simulink library "hamilton"  (R2023a)
settings: Solver=VariableStepAuto  StartTime=0.0  StopTime=10.0  RelTol=1e-3
undefined symbols (not defined in the file): b, d, g, J1, J2, J3, L, m
settings Model: Creator=Alex  LastModifiedBy=Alex

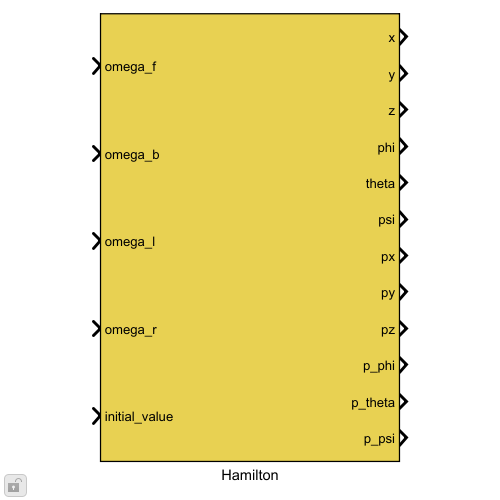
[thumbnail: Simulink's stored preview of the top-level diagram]
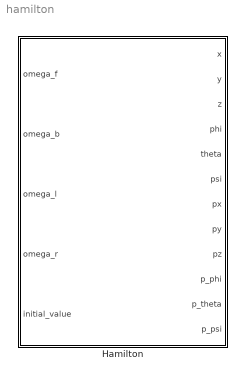
== system hamilton ==
  Hamilton : Subsystem

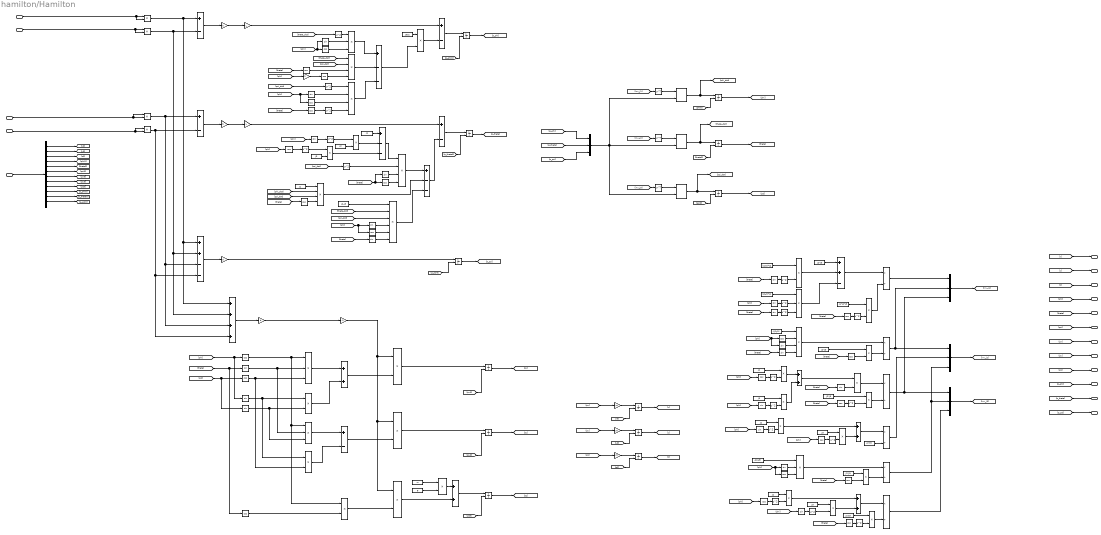
== system hamilton/Hamilton ==
  note: aefcascascxascx
  note: F_thrust
  note: Rotational generalized coordinates (positions)
  note: Translational generalized coordinates (positions)
  note: Translational momentum equations
  note: Rotational momentum equations
  note: Matrix J^(-1) computation
  omega_f : Inport
  omega_b : Inport  Port=2
  omega_l : Inport  Port=3
  omega_r : Inport  Port=4
  initial_value : Inport  Port=5
  Add{,1,3..4,11} (5 alike) : Sum  Inputs=+-
  Add{10,14,26..28} (5 alike) : Sum
  Add2 : Sum  Inputs=++--
  Add25 : Sum  Inputs=++-
  Add5 : Sum  Inputs=+--
  Add6 : Sum  Inputs=++++
  Add7 : Sum  Inputs=+--
  Add8 : Sum  Inputs=+--
  Constant1 : Constant  Value=J3-J2
  Constant2 : Constant  Value=J1
  Constant{22,26,28,31,34,36} (6 alike) : Constant  Value=J2*J3
  Constant23 : Constant  Value=(J1-J3)*J2
  Constant24 : Constant  Value=(J2-J3)*J1
  Constant25 : Constant  Value=J1*J2*J3
  Constant27 : Constant  Value=-(J2-J3)
  Constant{3,29,32,37} (4 alike) : Constant  Value=J2
  Constant{8,30,33,38} (4 alike) : Constant  Value=J3
  Constant35 : Constant  Value=-(J2-J3)
  Constant4 : Constant  Value=J1
  Constant5 : Constant  Value=J2-J3
  Constant6 : Constant  Value=m
  Constant7 : Constant  Value=g
  Cos{,1,3,5,7,53..55,58,60,63..64,66..67,69} (15 alike) : Trigonometry  Operator=cos
  Cos{4,6,8,50..52,56..57,59,61..62,65,68} (13 alike) : Trigonometry
  Demux : Demux  Outputs=12
  Divide{6..11} (6 alike) : Product  Inputs=*/
  Gain : Gain  Gain=b
  Gain1 : Gain  Gain=L
  Gain10 : Gain  Gain=-1
  Gain2 : Gain  Gain=b
  Gain3 : Gain  Gain=L
  Gain4 : Gain  Gain=d
  Gain5 : Gain  Gain=b
  Gain6 : Gain  Gain=1/m
  Gain7 : Gain  Gain=1/m
  Gain8 : Gain  Gain=1/m
  Gain9 : Gain  Gain=2
  Integrator{,1..11} (12 alike) : Integrator  InitialConditionSource=external
  Matrix Multiply1 : Product  Multiplication=Matrix(*)
  Matrix Multiply2 : Product  Multiplication=Matrix(*)
  Matrix Multiply5 : Product  Multiplication=Matrix(*)
  Mux{,7..9} (4 alike) : Mux  Inputs=3
  Product{,1..4,11..12,14,16..21,44,46..47,49..55,57..59} (27 alike) : Product
  Product10 : Product  Inputs=6
  Product{5,13,15,45,56} (5 alike) : Product  Inputs=3
  Product{6..9,48} (5 alike) : Product  Inputs=4
  Sin{,4,7..10} (6 alike) : Trigonometry
  Sin{1..3,5..6,11..12} (7 alike) : Trigonometry  Operator=cos
  Square{1..6,13..24} (18 alike) : Math  Operator=square
  Transpose1 : Math  Operator=transpose
  Transpose2 : Math  Operator=transpose
  Transpose5 : Math  Operator=transpose
  x : Outport
  y : Outport  Port=2
  z : Outport  Port=3
  phi : Outport  Port=4
  theta : Outport  Port=5
  psi : Outport  Port=6
  px : Outport  Port=7
  py : Outport  Port=8
  pz : Outport  Port=9
  p_phi : Outport  Port=10
  p_theta : Outport  Port=11
  p_psi : Outport  Port=12
  wires:
  omega_l/1 -> Product/2, Product/1
  omega_r/1 -> Product1/2, Product1/1
  Product/1 -> Add2/1, Add6/1, Add/1
  Product1/1 -> Add2/2, Add6/2, Add/2
  Add/1 -> Gain/1
  Gain/1 -> Gain1/1
  Gain1/1 -> Add3/1  "M1"
  Gain3/1 -> Add4/1  "M2"
  Gain2/1 -> Gain3/1
  Add1/1 -> Gain2/1
  Product3/1 -> Add6/4, Add2/4, Add1/2
  Product2/1 -> Add6/3, Add2/3, Add1/1
  omega_b/1 -> Product3/1, Product3/2
  omega_f/1 -> Product2/1, Product2/2
  Add2/1 -> Gain4/1
  Gain4/1 -> Integrator/1  "M3"
  Add6/1 -> Gain5/1
  Gain5/1 -> Gain10/1  "Fa"
  [phi] -> Sin9/1, Cos/1
  Cos/1 -> Product17/1, Product15/1, Product13/1
  [theta] -> Sin11/1, Sin8/1
  Sin8/1 -> Product15/2, Product13/2
  [psi] -> Cos1/1, Sin10/1
  Cos1/1 -> Product16/2, Product13/3
  Sin9/1 -> Product16/1, Product14/1
  Sin10/1 -> Product15/3, Product14/2
  Product13/1 -> Add10/1
  Product14/1 -> Add10/2
  Product15/1 -> Add11/1
  Product16/1 -> Add11/2
  Sin11/1 -> Product17/2
  Product17/1 -> Product20/2
  Add11/1 -> Product19/2
  Add10/1 -> Product18/2
  Product20/1 -> Add14/2
  Constant7/1 -> Product12/2
  Product18/1 -> Integrator6/1
  Integrator6/1 -> [px]  "px"
  Product19/1 -> Integrator7/1
  Integrator7/1 -> [py]  "py"
  Add14/1 -> Integrator8/1
  Integrator8/1 -> [pz]  "pz"
  [x] -> x/1
  [y] -> y/1
  [p_psi] -> p_psi/1
  [p_theta] -> p_theta/1
  [p_phi] -> p_phi/1
  [pz] -> pz/1
  [py] -> py/1
  [px] -> px/1
  [psi] -> psi/1
  [theta] -> theta/1
  [phi] -> phi/1
  [z] -> z/1
  Cos55/1 -> Product48/2
  Product46/1 -> Divide6/2
  [phi] -> Cos56/1, Cos55/1
  Square13/1 -> Product44/2
  Add27/1 -> Divide9/1
  Product57/1 -> Divide11/2
  [theta] -> Cos53/1
  Cos53/1 -> Square16/1
  [theta] -> Cos64/1
  Constant23/1 -> Product44/1
  Divide6/1 -> Mux7/1
  Cos58/1 -> Square17/1
  [theta] -> Cos58/1
  Mux7/1 -> [inv_j1]
  Product58/1 -> Add28/1
  Add28/1 -> Divide11/1
  Product59/1 -> Add28/2
  Cos57/1 -> Product48/4
  Add26/1 -> Product50/1
  Cos56/1 -> Product48/3
  Cos67/1 -> Square22/1
  Square22/1 -> Product57/2
  Mux8/1 -> [inv_j2]
  Divide11/1 -> Mux9/3
  Cos69/1 -> Square24/1
  Constant34/1 -> Product55/1
  [theta] -> Cos57/1
  Divide7/1 -> Mux8/1, Mux7/2
  Product52/1 -> Add26/1
  Constant22/1 -> Add25/1
  Constant36/1 -> Product57/1
  [theta] -> Cos50/1
  Constant26/1 -> Product47/1
  Constant35/1 -> Product56/1
  Add25/1 -> Divide6/1
  Cos66/1 -> Product56/3
  Product56/1 -> Divide10/1
  Cos65/1 -> Product56/2
  Cos63/1 -> Square21/1
  [phi] -> Cos61/1
  Constant25/1 -> Product46/1
  Square20/1 -> Product54/2
  Cos62/1 -> Square20/1
  Constant38/1 -> Product59/1
  Divide8/1 -> Mux9/1, Mux7/3
  Product53/1 -> Add27/2
  Product55/1 -> Divide10/2
  Square16/1 -> Product46/2
  Constant24/1 -> Product45/1
  Cos61/1 -> Square19/1
  Product44/1 -> Add25/2
  Square15/1 -> Product45/3
  Constant29/1 -> Product52/1
  Constant33/1 -> Product53/1
  Product51/1 -> Add26/2
  Product49/1 -> Divide8/2
  Product45/1 -> Add25/3
  Square19/1 -> Product51/2
  Constant28/1 -> Product49/1
  Constant32/1 -> Product54/1
  [theta] -> Cos52/1
  [phi] -> Cos68/1
  Cos68/1 -> Square23/1
  Cos51/1 -> Square14/1
  Square14/1 -> Product45/2
  Square18/1 -> Product52/2
  [theta] -> Cos59/1
  Cos54/1 -> Product47/2
  [theta] -> Cos54/1
  Constant31/1 -> Divide9/2
  Constant27/1 -> Product48/1
  Divide10/1 -> Mux9/2, Mux8/3
  [phi] -> Cos63/1
  [phi] -> Cos60/1
  Product54/1 -> Add27/1
  Cos64/1 -> Product55/2
  Constant30/1 -> Product51/1
  Mux9/1 -> [inv_j3]
  Square24/1 -> Product58/2
  Product50/1 -> Divide8/1
  [phi] -> Cos62/1
  Cos59/1 -> Product50/2
  Product47/1 -> Divide7/2
  Cos52/1 -> Square15/1
  [theta] -> Cos67/1
  Square17/1 -> Product49/2
  Product48/1 -> Divide7/1
  Cos50/1 -> Square13/1
  Square23/1 -> Product59/2
  Cos60/1 -> Square18/1
  Square21/1 -> Product53/2
  [phi] -> Cos69/1
  [phi] -> Cos66/1, Cos65/1
  Constant37/1 -> Product58/1
  Divide9/1 -> Mux8/2
  [phi] -> Cos51/1
  Integrator/1 -> [p_psi]
  Integrator1/1 -> [p_theta]
  Integrator2/1 -> [p_phi]
  Integrator4/1 -> [x]
  Integrator3/1 -> [y]
  Integrator5/1 -> [z]
  [px] -> Gain6/1
  Gain6/1 -> Integrator4/1
  [py] -> Gain7/1
  Gain7/1 -> Integrator3/1
  [pz] -> Gain8/1
  Gain8/1 -> Integrator5/1
  Integrator9/1 -> [phi]
  Integrator10/1 -> [theta]
  Integrator11/1 -> [psi]
  [p_phi] -> Mux/1
  [p_theta] -> Mux/2
  [p_psi] -> Mux/3
  Matrix Multiply5/1 -> [phi_dot], Integrator9/1
  Transpose5/1 -> Matrix Multiply5/1
  [inv_j1] -> Transpose5/1
  [inv_j2] -> Transpose1/1
  Transpose1/1 -> Matrix Multiply1/1
  Matrix Multiply1/1 -> [theta_dot], Integrator10/1
  Matrix Multiply2/1 -> [psi_dot], Integrator11/1
  [inv_j3] -> Transpose2/1
  Transpose2/1 -> Matrix Multiply2/1
  Mux/1 -> Matrix Multiply2/2, Matrix Multiply5/2, Matrix Multiply1/2
  Add4/1 -> Integrator1/1
  Add3/1 -> Integrator2/1
  Product4/1 -> Add3/2
  Constant1/1 -> Product4/1
  Add7/1 -> Product4/2
  Product5/1 -> Add7/1
  Product6/1 -> Add7/2
  Product7/1 -> Add7/3
  Add5/1 -> Add4/2
  Product8/1 -> Add5/1
  Product9/1 -> Add5/2
  Product10/1 -> Add5/3
  Add8/1 -> Product8/1
  Constant4/1 -> Product9/1
  Constant5/1 -> Product10/1
  [theta] -> Cos4/1, Cos3/1
  Cos3/1 -> Product8/4
  Cos4/1 -> Product8/3
  [theta_dot] -> Square1/1
  Square1/1 -> Product5/1
  [phi] -> Sin/1, Sin1/1
  Sin1/1 -> Product5/3
  Sin/1 -> Product5/2
  [theta_dot] -> Product6/1
  [psi_dot] -> Product6/2
  [theta] -> Sin2/1
  Sin2/1 -> Product6/3
  Sin3/1 -> Product6/4
  [phi] -> Gain9/1
  Gain9/1 -> Sin3/1
  Square2/1 -> Product7/1
  [psi_dot] -> Square2/1
  [phi] -> Sin4/1, Sin5/1
  Sin4/1 -> Product7/2
  Sin5/1 -> Product7/3
  [theta] -> Sin6/1
  Square3/1 -> Product7/4
  Sin6/1 -> Square3/1
  [psi_dot] -> Square4/1
  Square4/1 -> Product8/2
  [phi_dot] -> Product9/2
  [psi_dot] -> Product9/3
  [theta] -> Cos5/1
  Cos5/1 -> Product9/4
  [theta_dot] -> Product10/2
  [psi_dot] -> Product10/3
  [phi] -> Cos7/1, Cos6/1
  Cos6/1 -> Product10/4
  Cos7/1 -> Product10/5
  Cos8/1 -> Product10/6
  [theta] -> Cos8/1
  Gain10/1 -> Product20/1, Product19/1, Product18/1
  Product12/1 -> Add14/1
  Constant6/1 -> Product12/1
  Constant2/1 -> Add8/1
  Product11/1 -> Add8/2
  Product21/1 -> Add8/3
  Constant3/1 -> Product11/2
  Constant8/1 -> Product21/2
  [phi] -> Sin7/1
  Sin7/1 -> Square5/1
  Square5/1 -> Product11/1
  Sin12/1 -> Square6/1
  [phi] -> Sin12/1
  Square6/1 -> Product21/1
  Demux/3 -> [z0]
  Demux/9 -> [pz0]
  Demux/2 -> [y0]
  Demux/8 -> [py0]
  Demux/6 -> [psi0]
  Demux/7 -> [px0]
  Demux/5 -> [theta0]
  Demux/1 -> [x0]
  Demux/12 -> [p_psi0]
  initial_value/1 -> Demux/1
  Demux/10 -> [p_phi0]
  Demux/4 -> [phi0]
  Demux/11 -> [p_theta0]
  [z0] -> Integrator5/2
  [y0] -> Integrator3/2
  [x0] -> Integrator4/2
  [pz0] -> Integrator8/2
  [py0] -> Integrator7/2
  [px0] -> Integrator6/2
  [p_psi0] -> Integrator/2
  [p_theta0] -> Integrator1/2
  [p_phi0] -> Integrator2/2
  [phi0] -> Integrator9/2
  [theta0] -> Integrator10/2
  [psi0] -> Integrator11/2
